simulink model "controllo_cascata_nuovo"  (R2023b)
settings: Solver=VariableStepAuto  StartTime=0.0  StopTime=5  RelTol=1e-3
values from neighbouring files (symbols this model uses):
  C = 3212.6*(s+39.02)/(s+244.3)    [controllore_mag_lin.m]    (also in controllore_piu_anelli.m)
  den_mag_C = Gden{1}    [controllo_un_anello.m]    (also in controllore_cascata_nuovo.m)
  den_mag_M = Gden{1}    [controllo_un_anello.m]    (also in controllore_cascata_nuovo.m)
  ki = 2117.9265    [controllore_mag_lin.m]    (also in controllore_piu_anelli.m)
  kp = 46.0161    [controllore_mag_lin.m]    (also in controllore_piu_anelli.m)
  num_mag_C = Gnum{1}    [controllo_un_anello.m]    (also in controllore_cascata_nuovo.m)
  num_mag_M = Gnum{1}    [controllo_un_anello.m]    (also in controllore_cascata_nuovo.m)
  ueq = 15/Rtot    [controllore_mag_lin.m]    (also in controllore_piu_anelli.m)
  Veq = 12    [controllo_un_anello.m]    (also in controllore_cascata_nuovo.m)
undefined symbols (not defined in the file or in its folder): A, B, Lc, Rtot, x1_eq, y0
libraries: slpidlib x3
settings Model: Creator=lollo  LastModifiedBy=lollo

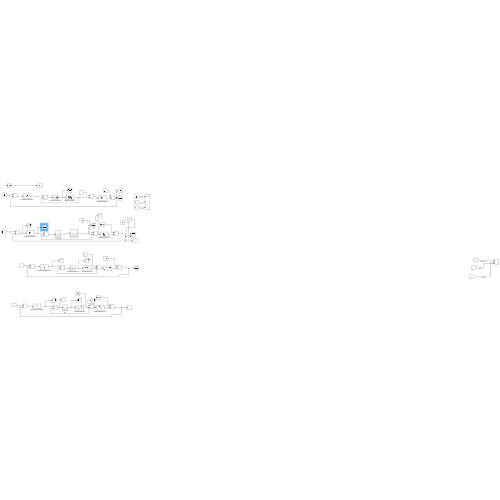
[thumbnail: Simulink's stored preview of the top-level diagram]
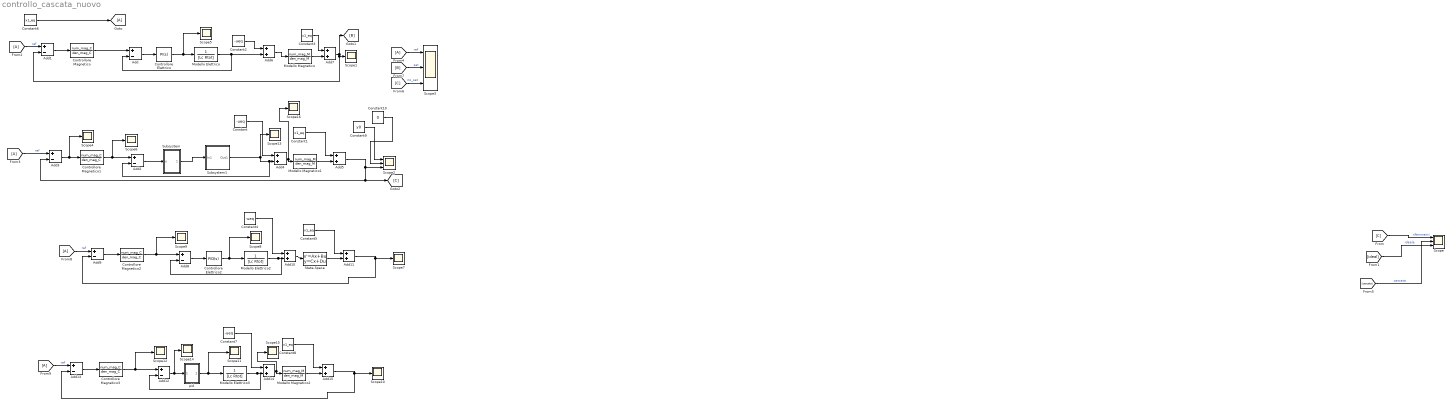
== system controllo_cascata_nuovo ==
  Add{,1..3,8..9,12..13} (8 alike) : Sum  Inputs=+-
  Add{4..7,10..11,14..15} (8 alike) : Sum
  Constant{,2,4,7} (4 alike) : Constant  Value=-ueq
  Constant{1,3,5..6,8} (5 alike) : Constant  Value=x1_eq
  Constant10 : Constant  Value=0
  Constant9 : Constant  Value=y0
  Controllore Elettrico : slpidlib/PID Controller  Controller=PI  Form=Parallel  TimeDomain=Continuous-time  UseExternalTs=off  SampleTime=-1  IntegratorMethod=Forward Euler  FilterMethod=Forward Euler  ControllerParametersSource=internal  P=kp  I=ki  UseKiTs=off  D=0  N=100  UseFilter=on  TunerSelectOption=Transfer Function Based (PID Tuner App)  InitialConditionSource=internal  InitialConditionForIntegrator=0  InitialConditionForFilter=0  DifferentiatorICPrevScaledInput=0  ExternalReset=none  TrackingMode=off  Kt=1  LimitOutput=on  SatLimitsSource=internal  UpperSaturationLimit=23  LowerSaturationLimit=-23  LinearizeAsGain=on  AntiWindupMode=clamping  Kb=1  LimitIntegrator=off  UpperIntegratorSaturationLimit=inf  LowerIntegratorSaturationLimit=-inf  POutMin=[]  POutMax=[]  IOutMin=[]  IOutMax=[]  DOutMin=[]  DOutMax=[]  NOutMin=[]  NOutMax=[]  SumOutMin=[]  SumOutMax=[]  SaturationOutMin=[]  SaturationOutMax=[]  PParamMin=[]  PParamMax=[]  IParamMin=[]  IParamMax=[]  DParamMin=[]  DParamMax=[]  NParamMin=[]  NParamMax=[]  KbParamMin=[]  KbParamMax=[]  KtParamMin=[]  KtParamMax=[]  KbOutMin=[]  KbOutMax=[]  KtOutMin=[]  KtOutMax=[]  IntegratorOutMin=[]  IntegratorOutMax=[]  FilterOutMin=[]  FilterOutMax=[]  SumI1OutMin=[]  SumI1OutMax=[]  SumI2OutMin=[]  SumI2OutMax=[]  SumI3OutMin=[]  SumI3OutMax=[]  SumI4OutMin=[]  SumI4OutMax=[]  SumDOutMin=[]  SumDOutMax=[]  DifferentiatorOutMin=[]  DifferentiatorOutMax=[]  FilterDiffOutCoefMin=[]  FilterDiffOutCoefMax=[]  ReciprocalOutMin=[]  ReciprocalOutMax=[]  SumDenOutMin=[]  SumDenOutMax=[]  SumNumOutMin=[]  SumNumOutMax=[]  DivideOutMin=[]  DivideOutMax=[]  UdiffTsProdOutMin=[]  UdiffTsProdOutMax=[]  NTsProdOutMin=[]  NTsProdOutMax=[]  UintegralTsProdOutMin=[]  UintegralTsProdOutMax=[]  UngainTsProdOutMin=[]  UngainTsProdOutMax=[]  ClampingZeroOutDataTypeStr=Inherit: Inherit via back propagation  ClampingZeroOutMin=[]  ClampingZeroOutMax=[]  FilterDenConstantOutDataTypeStr=Inherit: Inherit via back propagation  FilterDenConstantOutMin=[]  FilterDenConstantOutMax=[]  PCopyOutDataTypeStr=Inherit: Inherit via back propagation  PCopyOutMin=[]  PCopyOutMax=[]  NCopyOutDataTypeStr=Inherit: Inherit via back propagation  NCopyOutMin=[]  NCopyOutMax=[]  IntegratorContinuousStateAttributes=''  IntegratorStateMustResolveToSignalObject=off  IntegratorRTWStateStorageClass=Auto  FilterContinuousStateAttributes=''  FilterStateMustResolveToSignalObject=off  FilterRTWStateStorageClass=Auto  ParallelPVariant=InternalParameters  IdealPVariant=Disabled  IVariant=InternalParameters  DVariant=Disabled  IntegratorVariant=Continuous  SatVariant=Enabled  AWVariant=ContClampingParallel  PCopyVariant=Disabled  TRVariant=Disabled  FdbkBlocksVariant=Forward  IdealPFdbkVariant=Disabled  SatFdbkVariant=Disabled  DerivativeFilterVariant=Disabled  NVariant=Disabled  NCopyVariant=Disabled_SignalSpec  FilterICVariant=Disabled  IntegratorICVariant=InternalICs  ExternalResetVariant=Disabled  TRSumVariant=Passthrough  SumFdbkVariant=Disabled  SumVariant=Sum_PI  TsampFilterVariant=InternalTs  TsampNgainVariant=Passthrough  TsampIntegralVariant=Disabled_SignalSpec  ExternalSaturationOutDataTypeStr=Inherit: Same as second input
  Controllore Elettrico2 : slpidlib/PID Controller  Controller=PID  Form=Parallel  TimeDomain=Continuous-time  UseExternalTs=off  SampleTime=-1  IntegratorMethod=Forward Euler  FilterMethod=Forward Euler  ControllerParametersSource=internal  P=kp  I=ki  UseKiTs=off  D=0  N=100  UseFilter=on  TunerSelectOption=Transfer Function Based (PID Tuner App)  InitialConditionSource=internal  InitialConditionForIntegrator=0  InitialConditionForFilter=0  DifferentiatorICPrevScaledInput=0  ExternalReset=none  TrackingMode=off  Kt=1  LimitOutput=off  SatLimitsSource=internal  UpperSaturationLimit=23  LowerSaturationLimit=-23  LinearizeAsGain=on  AntiWindupMode=clamping  Kb=1  LimitIntegrator=off  UpperIntegratorSaturationLimit=inf  LowerIntegratorSaturationLimit=-inf  POutMin=[]  POutMax=[]  IOutMin=[]  IOutMax=[]  DOutMin=[]  DOutMax=[]  NOutMin=[]  NOutMax=[]  SumOutMin=[]  SumOutMax=[]  SaturationOutMin=[]  SaturationOutMax=[]  PParamMin=[]  PParamMax=[]  IParamMin=[]  IParamMax=[]  DParamMin=[]  DParamMax=[]  NParamMin=[]  NParamMax=[]  KbParamMin=[]  KbParamMax=[]  KtParamMin=[]  KtParamMax=[]  KbOutMin=[]  KbOutMax=[]  KtOutMin=[]  KtOutMax=[]  IntegratorOutMin=[]  IntegratorOutMax=[]  FilterOutMin=[]  FilterOutMax=[]  SumI1OutMin=[]  SumI1OutMax=[]  SumI2OutMin=[]  SumI2OutMax=[]  SumI3OutMin=[]  SumI3OutMax=[]  SumI4OutMin=[]  SumI4OutMax=[]  SumDOutMin=[]  SumDOutMax=[]  DifferentiatorOutMin=[]  DifferentiatorOutMax=[]  FilterDiffOutCoefMin=[]  FilterDiffOutCoefMax=[]  ReciprocalOutMin=[]  ReciprocalOutMax=[]  SumDenOutMin=[]  SumDenOutMax=[]  SumNumOutMin=[]  SumNumOutMax=[]  DivideOutMin=[]  DivideOutMax=[]  UdiffTsProdOutMin=[]  UdiffTsProdOutMax=[]  NTsProdOutMin=[]  NTsProdOutMax=[]  UintegralTsProdOutMin=[]  UintegralTsProdOutMax=[]  UngainTsProdOutMin=[]  UngainTsProdOutMax=[]  ClampingZeroOutDataTypeStr=Inherit: Inherit via back propagation  ClampingZeroOutMin=[]  ClampingZeroOutMax=[]  FilterDenConstantOutDataTypeStr=Inherit: Inherit via back propagation  FilterDenConstantOutMin=[]  FilterDenConstantOutMax=[]  PCopyOutDataTypeStr=Inherit: Inherit via back propagation  PCopyOutMin=[]  PCopyOutMax=[]  NCopyOutDataTypeStr=Inherit: Inherit via back propagation  NCopyOutMin=[]  NCopyOutMax=[]  IntegratorContinuousStateAttributes=''  IntegratorStateMustResolveToSignalObject=off  IntegratorRTWStateStorageClass=Auto  FilterContinuousStateAttributes=''  FilterStateMustResolveToSignalObject=off  FilterRTWStateStorageClass=Auto  ParallelPVariant=InternalParameters  IdealPVariant=Disabled  IVariant=InternalParameters  DVariant=InternalParameters  IntegratorVariant=Continuous  SatVariant=Disabled  AWVariant=Passthrough  PCopyVariant=Disabled  TRVariant=Disabled  FdbkBlocksVariant=Forward  IdealPFdbkVariant=Disabled  SatFdbkVariant=Disabled  DerivativeFilterVariant=ContFilter  NVariant=InternalParameters  NCopyVariant=Disabled  FilterICVariant=InternalICsFilter  IntegratorICVariant=InternalICs  ExternalResetVariant=Disabled  TRSumVariant=Passthrough  SumFdbkVariant=Disabled  SumVariant=Sum_PID  TsampFilterVariant=InternalTs  TsampNgainVariant=Passthrough  TsampIntegralVariant=Disabled_SignalSpec  ExternalSaturationOutDataTypeStr=Inherit: Same as second input
  Controllore Magnetico{,1..3} (4 alike) : TransferFcn  Numerator=num_mag_C  Denominator=den_mag_C
  From{2..4,8..9} (5 alike) : From
  Goto : Goto
  Modello Elettrico : TransferFcn  Denominator=[Lc Rtot]
  Modello Elettrico2 : TransferFcn  Denominator=[Lc Rtot]
  Modello Elettrico3 : TransferFcn  Denominator=[Lc Rtot]
  Modello Magnetico : TransferFcn  Numerator=num_mag_M  Denominator=den_mag_M
  Modello Magnetico1 : TransferFcn  Numerator=num_mag_M  Denominator=den_mag_M
  Modello Magnetico2 : TransferFcn  Numerator=num_mag_M  Denominator=den_mag_M
  Scope : Scope  NumInputPorts=3
  Scope{1,4..16} (14 alike) : Scope
  Scope2 : Scope  NumInputPorts=3
  Scope3 : Scope  NumInputPorts=3
  State-Space : StateSpace  A=A  B=B  C=C  D=0  InitialCondition=0.001
  Subsystem : Subsystem
  Subsystem1 : Subsystem
  pid : Subsystem
  wires:
  [C] -> Scope/1  "riferimenti"
  [ideal] -> Scope/3  "ideale"
  [cascata] -> Scope/2  "cascata"
  Controllore Elettrico/1 -> Scope5/1, Modello Elettrico/1
  Modello Elettrico/1 -> Add6/2, Add/2
  Add/1 -> Controllore Elettrico/1
  Controllore Magnetico/1 -> Add/1
  Add1/1 -> Controllore Magnetico/1
  From2/1 -> Add1/1  "ref"
  Add3/1 -> Scope4/1, Controllore Magnetico1/1
  From3/1 -> Add3/1  "ref"
  Controllore Magnetico1/1 -> Add2/1, Scope6/1
  From4/1 -> Scope3/1  "ref"
  [B] -> Scope3/2  "sat"
  [C] -> Scope3/3  "no_sat"
  Add4/1 -> Modello Magnetico1/1, Scope16/1
  Constant/1 -> Add4/1
  Constant1/1 -> Add5/1
  Modello Magnetico1/1 -> Add5/2
  Add5/1 -> Add3/2, [C], Scope2/3
  Add6/1 -> Modello Magnetico/1
  Constant2/1 -> Add6/1
  Add7/1 -> Add1/2, Scope1/1, [B]
  Modello Magnetico/1 -> Add7/2
  Constant3/1 -> Add7/1
  Constant5/1 -> Add11/1
  Add11/1 -> Add9/2, Scope7/1
  State-Space/1 -> Add11/2
  Constant4/1 -> Add10/1
  Add10/1 -> State-Space/1
  From8/1 -> Add9/1  "ref"
  Controllore Magnetico2/1 -> Scope9/1, Add8/1
  Add8/1 -> Controllore Elettrico2/1
  Add9/1 -> Controllore Magnetico2/1
  Controllore Elettrico2/1 -> Scope8/1, Modello Elettrico2/1
  Modello Elettrico2/1 -> Add8/2, Add10/2
  Constant6/1 -> Goto/1
  Modello Magnetico2/1 -> Add15/2
  Add15/1 -> Add13/2, Scope10/1
  Controllore Magnetico3/1 -> Scope12/1, Add12/1
  Constant7/1 -> Add14/1
  Add12/1 -> Scope14/1, pid/1(In1)
  pid/1(Out1) -> Scope11/1, Modello Elettrico3/1
  Modello Elettrico3/1 -> Add12/2, Add14/2
  From9/1 -> Add13/1  "ref"
  Add13/1 -> Controllore Magnetico3/1
  Constant8/1 -> Add15/1
  Add14/1 -> Scope15/1, Modello Magnetico2/1
  Add2/1 -> Subsystem/1(u)
  Subsystem1/1(Out1) -> Add2/2, Add4/2, Scope13/1
  Subsystem/1(Out1) -> Subsystem1/1(In1)
  Constant9/1 -> Scope2/1
  Constant10/1 -> Scope2/2

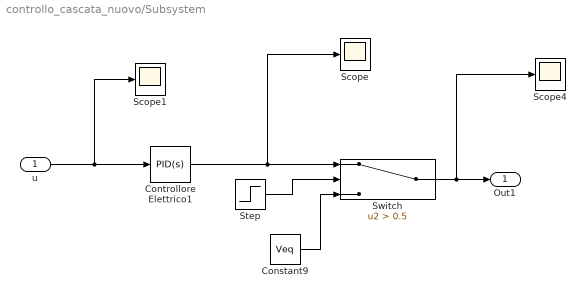
== system controllo_cascata_nuovo/Subsystem ==
  u : Inport
  Constant9 : Constant  Value=Veq
  Controllore Elettrico1 : slpidlib/PID Controller  Controller=PID  Form=Parallel  TimeDomain=Continuous-time  UseExternalTs=off  SampleTime=-1  IntegratorMethod=Forward Euler  FilterMethod=Forward Euler  ControllerParametersSource=internal  P=kp  I=ki  UseKiTs=off  D=0  N=100  UseFilter=on  TunerSelectOption=Transfer Function Based (PID Tuner App)  InitialConditionSource=internal  InitialConditionForIntegrator=0  InitialConditionForFilter=0  DifferentiatorICPrevScaledInput=0  ExternalReset=none  TrackingMode=off  Kt=1  LimitOutput=off  SatLimitsSource=internal  UpperSaturationLimit=23  LowerSaturationLimit=-23  LinearizeAsGain=on  AntiWindupMode=clamping  Kb=1  LimitIntegrator=off  UpperIntegratorSaturationLimit=inf  LowerIntegratorSaturationLimit=-inf  POutMin=[]  POutMax=[]  IOutMin=[]  IOutMax=[]  DOutMin=[]  DOutMax=[]  NOutMin=[]  NOutMax=[]  SumOutMin=[]  SumOutMax=[]  SaturationOutMin=[]  SaturationOutMax=[]  PParamMin=[]  PParamMax=[]  IParamMin=[]  IParamMax=[]  DParamMin=[]  DParamMax=[]  NParamMin=[]  NParamMax=[]  KbParamMin=[]  KbParamMax=[]  KtParamMin=[]  KtParamMax=[]  KbOutMin=[]  KbOutMax=[]  KtOutMin=[]  KtOutMax=[]  IntegratorOutMin=[]  IntegratorOutMax=[]  FilterOutMin=[]  FilterOutMax=[]  SumI1OutMin=[]  SumI1OutMax=[]  SumI2OutMin=[]  SumI2OutMax=[]  SumI3OutMin=[]  SumI3OutMax=[]  SumI4OutMin=[]  SumI4OutMax=[]  SumDOutMin=[]  SumDOutMax=[]  DifferentiatorOutMin=[]  DifferentiatorOutMax=[]  FilterDiffOutCoefMin=[]  FilterDiffOutCoefMax=[]  ReciprocalOutMin=[]  ReciprocalOutMax=[]  SumDenOutMin=[]  SumDenOutMax=[]  SumNumOutMin=[]  SumNumOutMax=[]  DivideOutMin=[]  DivideOutMax=[]  UdiffTsProdOutMin=[]  UdiffTsProdOutMax=[]  NTsProdOutMin=[]  NTsProdOutMax=[]  UintegralTsProdOutMin=[]  UintegralTsProdOutMax=[]  UngainTsProdOutMin=[]  UngainTsProdOutMax=[]  ClampingZeroOutDataTypeStr=Inherit: Inherit via back propagation  ClampingZeroOutMin=[]  ClampingZeroOutMax=[]  FilterDenConstantOutDataTypeStr=Inherit: Inherit via back propagation  FilterDenConstantOutMin=[]  FilterDenConstantOutMax=[]  PCopyOutDataTypeStr=Inherit: Inherit via back propagation  PCopyOutMin=[]  PCopyOutMax=[]  NCopyOutDataTypeStr=Inherit: Inherit via back propagation  NCopyOutMin=[]  NCopyOutMax=[]  IntegratorContinuousStateAttributes=''  IntegratorStateMustResolveToSignalObject=off  IntegratorRTWStateStorageClass=Auto  FilterContinuousStateAttributes=''  FilterStateMustResolveToSignalObject=off  FilterRTWStateStorageClass=Auto  ParallelPVariant=InternalParameters  IdealPVariant=Disabled  IVariant=InternalParameters  DVariant=InternalParameters  IntegratorVariant=Continuous  SatVariant=Disabled  AWVariant=Passthrough  PCopyVariant=Disabled  TRVariant=Disabled  FdbkBlocksVariant=Forward  IdealPFdbkVariant=Disabled  SatFdbkVariant=Disabled  DerivativeFilterVariant=ContFilter  NVariant=InternalParameters  NCopyVariant=Disabled  FilterICVariant=InternalICsFilter  IntegratorICVariant=InternalICs  ExternalResetVariant=Disabled  TRSumVariant=Passthrough  SumFdbkVariant=Disabled  SumVariant=Sum_PID  TsampFilterVariant=InternalTs  TsampNgainVariant=Passthrough  TsampIntegralVariant=Disabled_SignalSpec  ExternalSaturationOutDataTypeStr=Inherit: Same as second input
  Scope : Scope
  Scope1 : Scope
  Scope4 : Scope
  Step : Step  Time=0.1  SampleTime=0
  Switch : Switch  Criteria=u2 > Threshold  Threshold=0.5  SaturateOnIntegerOverflow=off  InputSameDT=off
  Out1 : Outport
  wires:
  Controllore Elettrico1/1 -> Scope/1, Switch/1
  Constant9/1 -> Switch/3
  Switch/1 -> Scope4/1, Out1/1
  Step/1 -> Switch/2
  u/1 -> Scope1/1, Controllore Elettrico1/1

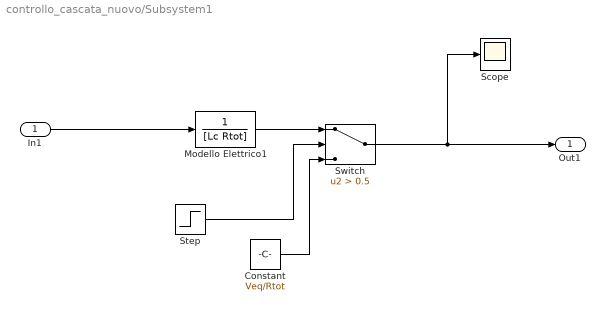
== system controllo_cascata_nuovo/Subsystem1 ==
  In1 : Inport
  Constant : Constant  Value=Veq/Rtot
  Modello Elettrico1 : TransferFcn  Denominator=[Lc Rtot]
  Scope : Scope
  Step : Step  Time=0.1  SampleTime=0
  Switch : Switch  Criteria=u2 > Threshold  Threshold=0.5  SaturateOnIntegerOverflow=off  InputSameDT=off
  Out1 : Outport
  wires:
  Modello Elettrico1/1 -> Switch/1
  In1/1 -> Modello Elettrico1/1
  Switch/1 -> Scope/1, Out1/1
  Step/1 -> Switch/2
  Constant/1 -> Switch/3

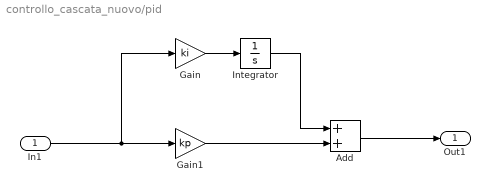
== system controllo_cascata_nuovo/pid ==
  In1 : Inport
  Add : Sum
  Gain : Gain  Gain=ki
  Gain1 : Gain  Gain=kp
  Integrator : Integrator
  Out1 : Outport
  wires:
  In1/1 -> Gain/1, Gain1/1
  Gain/1 -> Integrator/1
  Integrator/1 -> Add/1
  Gain1/1 -> Add/2
  Add/1 -> Out1/1
